simulink model "guidance"  (R2022b)
settings: Solver=ode4  StartTime=0.0  StopTime=1000  FixedStep=tims_sampling  RelTol=1e-3
values from neighbouring files (symbols this model uses):
  gamma0 = pi / 4    (= 0.785398163397)    [guidance_script.m]
  k = 4    [guidance_script.m]
  L = 0.729321661910    (= 0.72932166191)    [guidance_script.m]
  motor2steer_ratio = 33 / 60    (= 0.55)    [guidance_script.m]
  tau = 0.1    [guidance_script.m]
  V = 3    [guidance_script.m]
  x0 = 0    [guidance_script.m]
  xt = 10    [guidance_script.m]
  y0 = 0    [guidance_script.m]
  yt = 0    [guidance_script.m]
settings Model: Creator=jarry_goon  LastModifiedBy=jarry_goon

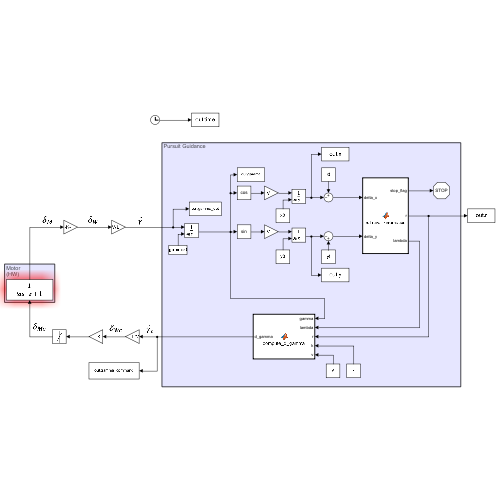
[thumbnail: Simulink's stored preview of the top-level diagram]
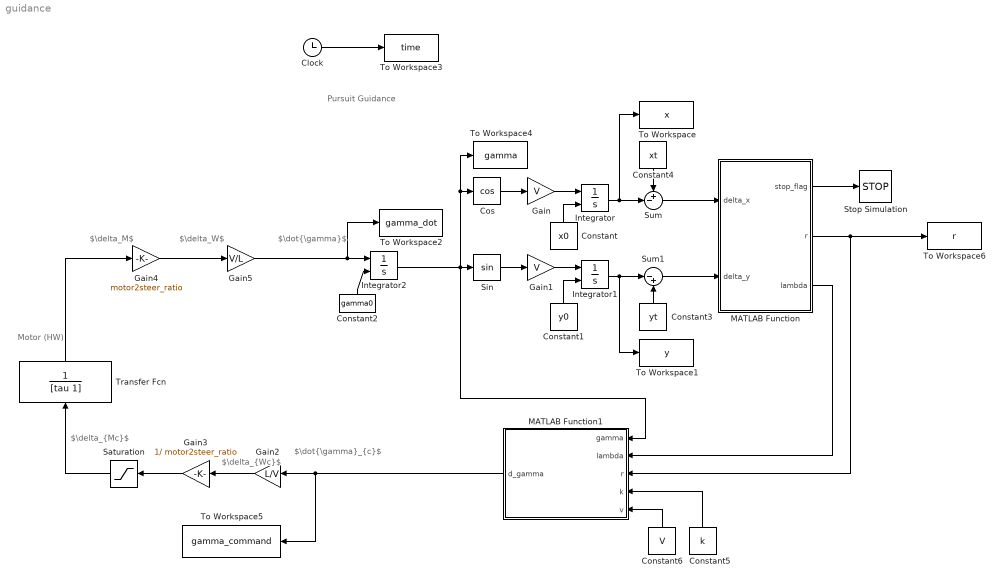
== system guidance ==
  note: $\dot{\gamma}_{c}$
  note: Motor
      | (HW)
  note: Pursuit Guidance
  note: $\delta_M$
  note: $\delta_{Wc}$
  note: $\delta_{Mc}$
  note: $\delta_W$
  note: $\dot{\gamma}$
  Clock : Clock
  Constant : Constant  Value=x0
  Constant1 : Constant  Value=y0
  Constant2 : Constant  Value=gamma0
  Constant3 : Constant  Value=yt
  Constant4 : Constant  Value=xt
  Constant5 : Constant  Value=k
  Constant6 : Constant  Value=V
  Cos : Trigonometry  Operator=cos
  Gain : Gain  Gain=V
  Gain1 : Gain  Gain=V
  Gain2 : Gain  Gain=L/V
  Gain3 : Gain  Gain=1/ motor2steer_ratio
  Gain4 : Gain  Gain=motor2steer_ratio
  Gain5 : Gain  Gain=V/L
  Integrator : Integrator  InitialConditionSource=external
  Integrator1 : Integrator  InitialConditionSource=external
  Integrator2 : Integrator  InitialConditionSource=external
  MATLAB Function : MATLAB Function  TreatAsAtomicUnit=on
  MATLAB Function1 : MATLAB Function  TreatAsAtomicUnit=on
  Saturation : Saturate  UpperLimit=pi / 3  LowerLimit=-pi / 3
  Sin : Trigonometry
  Stop Simulation : Stop
  Sum : Sum  Inputs=+-|
  Sum1 : Sum  Inputs=|-+
  To Workspace : ToWorkspace  VariableName=x  SampleTime=-1
      settings: Save2DSignal=2-D array (concatenate along first dimension)
  To Workspace1 : ToWorkspace  VariableName=y  SampleTime=-1
      settings: Save2DSignal=2-D array (concatenate along first dimension)
  To Workspace2 : ToWorkspace  VariableName=gamma_dot  SampleTime=-1
      settings: Save2DSignal=2-D array (concatenate along first dimension)
  To Workspace3 : ToWorkspace  VariableName=time  SampleTime=-1
      settings: Save2DSignal=2-D array (concatenate along first dimension)
  To Workspace4 : ToWorkspace  VariableName=gamma  SampleTime=-1
      settings: Save2DSignal=2-D array (concatenate along first dimension)
  To Workspace5 : ToWorkspace  VariableName=gamma_command  SampleTime=-1
      settings: Save2DSignal=2-D array (concatenate along first dimension)
  To Workspace6 : ToWorkspace  VariableName=r  SampleTime=-1
      settings: Save2DSignal=2-D array (concatenate along first dimension)
  Transfer Fcn : TransferFcn  Denominator=[tau 1]
  wires:
  Constant/1 -> Integrator/2
  Constant1/1 -> Integrator1/2
  Cos/1 -> Gain/1
  Sin/1 -> Gain1/1
  Constant2/1 -> Integrator2/2
  Integrator1/1 -> To Workspace1/1, Sum1/1
  Integrator/1 -> To Workspace/1, Sum/2
  Constant3/1 -> Sum1/2
  Constant4/1 -> Sum/1
  Sum/1 -> MATLAB Function/1(delta_x)
  Sum1/1 -> MATLAB Function/2(delta_y)
  MATLAB Function/2(r) -> MATLAB Function1/3(r), To Workspace6/1
  MATLAB Function/3(lambda) -> MATLAB Function1/2(lambda)
  Constant5/1 -> MATLAB Function1/4(k)
  Constant6/1 -> MATLAB Function1/5(v)
  Gain/1 -> Integrator/1
  Gain1/1 -> Integrator1/1
  MATLAB Function/1(stop_flag) -> Stop Simulation/1
  Clock/1 -> To Workspace3/1
  Integrator2/1 -> MATLAB Function1/1(gamma), Cos/1, To Workspace4/1, Sin/1
  MATLAB Function1/1(d_gamma) -> To Workspace5/1, Gain2/1
  Gain2/1 -> Gain3/1
  Gain3/1 -> Saturation/1
  Saturation/1 -> Transfer Fcn/1
  Transfer Fcn/1 -> Gain4/1
  Gain4/1 -> Gain5/1
  Gain5/1 -> Integrator2/1, To Workspace2/1

== matlab function guidance/MATLAB Function1 ==
  data: gamma input; lambda input; r input; d_gamma output; k input; v input
function d_gamma = compute_d_gamma(gamma, lambda, r, k, v)

d_gamma = - k * v / r * sin(gamma - lambda);

== matlab function guidance/MATLAB Function ==
  data: stop_flag output; delta_x input; r output; delta_y input; lambda output
function [stop_flag, r, lambda]= relative_kinematics(delta_x, delta_y)

tol = 0.2;

if(abs(delta_x) < tol && abs(delta_y) < tol)
    stop_flag = 1;
else
    stop_flag = 0;
end

r = sqrt(delta_x * delta_x + delta_y * delta_y);

lambda = atan2(delta_y, delta_x);
